simulink model "LC62_PIDControl_V6"  (R2022b)
settings: Solver=ode4  StartTime=0.0  StopTime=SimTime  FixedStep=1/500  RelTol=1e-3
model workspace (MAT data in the model file):
  Tr = 0.1
  freq = 0.002
  hover_w = 0.55
values from neighbouring files (symbols this model uses):
  b = 1.1    [initfun.m]
  c = 0.551    [initfun.m]
  Cll_beta = -0.0518    [initfun.m]
  Cll_del_A = -0.0369 * 5    (= -0.1845)    [initfun.m]
  Cll_del_R = 0.0026    [initfun.m]
  Cll_p = -0.4624    [initfun.m]
  Cll_r = 0.0218    [initfun.m]
  Cm_del_A = 0.001156    [initfun.m]
  Cm_del_E = -0.676    [initfun.m]
  Cn_beta = 0.0866    [initfun.m]
  Cn_del_A = -0.000385    [initfun.m]
  Cn_del_R = -0.0190    (= -0.019)    [initfun.m]
  Cn_p = -0.0048    [initfun.m]
  Cn_r = -0.0723    [initfun.m]
  Cy_beta = -1.1269    [initfun.m]
  Cy_del_R = 0.0534    [initfun.m]
  Cy_p = 0.0    (= 0)    [initfun.m]
  Cy_r = 0.2374    [initfun.m]
  d = 0.849    [initfun.m]
  dx1 = 0.9325+0.049    (= 0.9815)    [initfun.m]
  dx2 = 0.0725-0.049    (= 0.0235)    [initfun.m]
  dx3 = 1.1725-0.049    (= 1.1235)    [initfun.m]
  dy1 = 0.717 + temp_y    (= 0.717)    [initfun.m]
  dy2 = 0.717 - temp_y    (= 0.717)    [initfun.m]
  g = 9.81    [initfun.m]
  m = 41.97    [initfun.m]
  S = S1 + S2    (= 0.8522)    [initfun.m]
  S2 = 0.5898    [initfun.m]
undefined symbols (not defined in the file or in its folder): d2r, Earth, F, Light, MIL, sigbuilder_block, WGS84
libraries: simulink_extras x50, slpidlib x14, simulink x11, dspstat3 x5, aerolibwind2 x3, sharedTrackingLibrary x2, aerolibasang x2, aerolibtransform2 x2, robotcorelib x1, uavutilslib x1, uavalgslib x1, aerolibnav x1
(part 3 of 4)

== system LC62_PIDControl_V6/Position and Acceleration Control/Position Control ==
  note: [ States ]
      | u v w [m/s]
      | phi theta psi [rad]
      | p q r [rad/s]
      | X Y Z [m]
      | U V W [m/s]
  Position cmd : Inport
  States : Inport  Port=2
  Add : Sum  Inputs=+-
  Demux : Demux  Outputs=3
  Mux : Mux  Inputs=3
  PID_X : slpidlib/PID Controller  Controller=PID  Form=Parallel  TimeDomain=Discrete-time  UseExternalTs=off  SampleTime=-1  IntegratorMethod=Forward Euler  FilterMethod=Forward Euler  ControllerParametersSource=internal  P=0.45  I=0.005  UseKiTs=off  D=0.8  N=100  UseFilter=on  TunerSelectOption=Transfer Function Based (PID Tuner App)  InitialConditionSource=internal  InitialConditionForIntegrator=0  InitialConditionForFilter=0  DifferentiatorICPrevScaledInput=0  ExternalReset=none  TrackingMode=off  Kt=1  LimitOutput=on  SatLimitsSource=internal  UpperSaturationLimit=3  LowerSaturationLimit=-3  LinearizeAsGain=on  AntiWindupMode=clamping  Kb=1  LimitIntegrator=off  UpperIntegratorSaturationLimit=inf  LowerIntegratorSaturationLimit=-inf  POutMin=[]  POutMax=[]  IOutMin=[]  IOutMax=[]  DOutMin=[]  DOutMax=[]  NOutMin=[]  NOutMax=[]  SumOutMin=[]  SumOutMax=[]  SaturationOutMin=[]  SaturationOutMax=[]  PParamMin=[]  PParamMax=[]  IParamMin=[]  IParamMax=[]  DParamMin=[]  DParamMax=[]  NParamMin=[]  NParamMax=[]  KbParamMin=[]  KbParamMax=[]  KtParamMin=[]  KtParamMax=[]  KbOutMin=[]  KbOutMax=[]  KtOutMin=[]  KtOutMax=[]  IntegratorOutMin=[]  IntegratorOutMax=[]  FilterOutMin=[]  FilterOutMax=[]  SumI1OutMin=SumI1OutMin  SumI1OutMax=SumI1OutMax  SumI2OutMin=[]  SumI2OutMax=[]  SumI3OutMin=[]  SumI3OutMax=[]  SumI4OutMin=[]  SumI4OutMax=[]  SumDOutMin=[]  SumDOutMax=[]  DifferentiatorOutMin=[]  DifferentiatorOutMax=[]  FilterDiffOutCoefMin=[]  FilterDiffOutCoefMax=[]  ReciprocalOutMin=[]  ReciprocalOutMax=[]  SumDenOutMin=[]  SumDenOutMax=[]  SumNumOutMin=[]  SumNumOutMax=[]  DivideOutMin=[]  DivideOutMax=[]  UdiffTsProdOutMin=[]  UdiffTsProdOutMax=[]  NTsProdOutMin=[]  NTsProdOutMax=[]  UintegralTsProdOutMin=[]  UintegralTsProdOutMax=[]  UngainTsProdOutMin=[]  UngainTsProdOutMax=[]  ClampingZeroOutDataTypeStr=Inherit: Inherit via back propagation  ClampingZeroOutMin=[]  ClampingZeroOutMax=[]  FilterDenConstantOutDataTypeStr=Inherit: Inherit via back propagation  FilterDenConstantOutMin=[]  FilterDenConstantOutMax=[]  PCopyOutDataTypeStr=Inherit: Inherit via back propagation  PCopyOutMin=[]  PCopyOutMax=[]  NCopyOutDataTypeStr=Inherit: Inherit via back propagation  NCopyOutMin=[]  NCopyOutMax=[]  IntegratorContinuousStateAttributes=''  IntegratorStateMustResolveToSignalObject=off  IntegratorRTWStateStorageClass=Auto  FilterContinuousStateAttributes=''  FilterStateMustResolveToSignalObject=off  FilterRTWStateStorageClass=Auto  ParallelPVariant=InternalParameters  IdealPVariant=Disabled  IVariant=InternalParameters  DVariant=InternalParameters  IntegratorVariant=Discrete  SatVariant=Enabled  AWVariant=DiscClampingParallel  PCopyVariant=Disabled  TRVariant=Disabled  FdbkBlocksVariant=Forward  IdealPFdbkVariant=Disabled  SatFdbkVariant=Disabled  DerivativeFilterVariant=ForwardEulerFilter  NVariant=InternalParameters  NCopyVariant=Disabled  FilterICVariant=InternalICsFilter  IntegratorICVariant=InternalICs  ExternalResetVariant=Disabled  TRSumVariant=Passthrough  SumFdbkVariant=Disabled  SumVariant=Sum_PID  TsampFilterVariant=InternalTs  TsampNgainVariant=Passthrough  TsampIntegralVariant=Passthrough  ExternalSaturationOutDataTypeStr=Inherit: Same as second input
      settings: AttributesFormatString=P: %<P>, I: %<I>, D:%<D>
  PID_Y : slpidlib/PID Controller  Controller=PID  Form=Parallel  TimeDomain=Discrete-time  UseExternalTs=off  SampleTime=-1  IntegratorMethod=Forward Euler  FilterMethod=Forward Euler  ControllerParametersSource=internal  P=0.45  I=0.005  UseKiTs=off  D=0.8  N=100  UseFilter=on  TunerSelectOption=Transfer Function Based (PID Tuner App)  InitialConditionSource=internal  InitialConditionForIntegrator=0  InitialConditionForFilter=0  DifferentiatorICPrevScaledInput=0  ExternalReset=none  TrackingMode=off  Kt=1  LimitOutput=on  SatLimitsSource=internal  UpperSaturationLimit=3  LowerSaturationLimit=-3  LinearizeAsGain=on  AntiWindupMode=clamping  Kb=1  LimitIntegrator=off  UpperIntegratorSaturationLimit=inf  LowerIntegratorSaturationLimit=-inf  POutMin=[]  POutMax=[]  IOutMin=[]  IOutMax=[]  DOutMin=[]  DOutMax=[]  NOutMin=[]  NOutMax=[]  SumOutMin=[]  SumOutMax=[]  SaturationOutMin=[]  SaturationOutMax=[]  PParamMin=[]  PParamMax=[]  IParamMin=[]  IParamMax=[]  DParamMin=[]  DParamMax=[]  NParamMin=[]  NParamMax=[]  KbParamMin=[]  KbParamMax=[]  KtParamMin=[]  KtParamMax=[]  KbOutMin=[]  KbOutMax=[]  KtOutMin=[]  KtOutMax=[]  IntegratorOutMin=[]  IntegratorOutMax=[]  FilterOutMin=[]  FilterOutMax=[]  SumI1OutMin=SumI1OutMin  SumI1OutMax=SumI1OutMax  SumI2OutMin=[]  SumI2OutMax=[]  SumI3OutMin=[]  SumI3OutMax=[]  SumI4OutMin=[]  SumI4OutMax=[]  SumDOutMin=[]  SumDOutMax=[]  DifferentiatorOutMin=[]  DifferentiatorOutMax=[]  FilterDiffOutCoefMin=[]  FilterDiffOutCoefMax=[]  ReciprocalOutMin=[]  ReciprocalOutMax=[]  SumDenOutMin=[]  SumDenOutMax=[]  SumNumOutMin=[]  SumNumOutMax=[]  DivideOutMin=[]  DivideOutMax=[]  UdiffTsProdOutMin=[]  UdiffTsProdOutMax=[]  NTsProdOutMin=[]  NTsProdOutMax=[]  UintegralTsProdOutMin=[]  UintegralTsProdOutMax=[]  UngainTsProdOutMin=[]  UngainTsProdOutMax=[]  ClampingZeroOutDataTypeStr=Inherit: Inherit via back propagation  ClampingZeroOutMin=[]  ClampingZeroOutMax=[]  FilterDenConstantOutDataTypeStr=Inherit: Inherit via back propagation  FilterDenConstantOutMin=[]  FilterDenConstantOutMax=[]  PCopyOutDataTypeStr=Inherit: Inherit via back propagation  PCopyOutMin=[]  PCopyOutMax=[]  NCopyOutDataTypeStr=Inherit: Inherit via back propagation  NCopyOutMin=[]  NCopyOutMax=[]  IntegratorContinuousStateAttributes=''  IntegratorStateMustResolveToSignalObject=off  IntegratorRTWStateStorageClass=Auto  FilterContinuousStateAttributes=''  FilterStateMustResolveToSignalObject=off  FilterRTWStateStorageClass=Auto  ParallelPVariant=InternalParameters  IdealPVariant=Disabled  IVariant=InternalParameters  DVariant=InternalParameters  IntegratorVariant=Discrete  SatVariant=Enabled  AWVariant=DiscClampingParallel  PCopyVariant=Disabled  TRVariant=Disabled  FdbkBlocksVariant=Forward  IdealPFdbkVariant=Disabled  SatFdbkVariant=Disabled  DerivativeFilterVariant=ForwardEulerFilter  NVariant=InternalParameters  NCopyVariant=Disabled  FilterICVariant=InternalICsFilter  IntegratorICVariant=InternalICs  ExternalResetVariant=Disabled  TRSumVariant=Passthrough  SumFdbkVariant=Disabled  SumVariant=Sum_PID  TsampFilterVariant=InternalTs  TsampNgainVariant=Passthrough  TsampIntegralVariant=Passthrough  ExternalSaturationOutDataTypeStr=Inherit: Same as second input
      settings: AttributesFormatString=P: %<P>, I: %<I>, D:%<D>
  PID_Z : slpidlib/PID Controller  Controller=PID  Form=Parallel  TimeDomain=Discrete-time  UseExternalTs=off  SampleTime=-1  IntegratorMethod=Forward Euler  FilterMethod=Forward Euler  ControllerParametersSource=internal  P=6.8  I=0  UseKiTs=off  D=2.5  N=14.495  UseFilter=on  TunerSelectOption=Transfer Function Based (PID Tuner App)  InitialConditionSource=internal  InitialConditionForIntegrator=0  InitialConditionForFilter=0  DifferentiatorICPrevScaledInput=0  ExternalReset=none  TrackingMode=off  Kt=1  LimitOutput=on  SatLimitsSource=internal  UpperSaturationLimit=3  LowerSaturationLimit=-3  LinearizeAsGain=on  AntiWindupMode=clamping  Kb=1  LimitIntegrator=off  UpperIntegratorSaturationLimit=inf  LowerIntegratorSaturationLimit=-inf  POutMin=[]  POutMax=[]  IOutMin=[]  IOutMax=[]  DOutMin=[]  DOutMax=[]  NOutMin=[]  NOutMax=[]  SumOutMin=[]  SumOutMax=[]  SaturationOutMin=[]  SaturationOutMax=[]  PParamMin=[]  PParamMax=[]  IParamMin=[]  IParamMax=[]  DParamMin=[]  DParamMax=[]  NParamMin=[]  NParamMax=[]  KbParamMin=[]  KbParamMax=[]  KtParamMin=[]  KtParamMax=[]  KbOutMin=[]  KbOutMax=[]  KtOutMin=[]  KtOutMax=[]  IntegratorOutMin=[]  IntegratorOutMax=[]  FilterOutMin=[]  FilterOutMax=[]  SumI1OutMin=SumI1OutMin  SumI1OutMax=SumI1OutMax  SumI2OutMin=[]  SumI2OutMax=[]  SumI3OutMin=[]  SumI3OutMax=[]  SumI4OutMin=[]  SumI4OutMax=[]  SumDOutMin=[]  SumDOutMax=[]  DifferentiatorOutMin=[]  DifferentiatorOutMax=[]  FilterDiffOutCoefMin=[]  FilterDiffOutCoefMax=[]  ReciprocalOutMin=[]  ReciprocalOutMax=[]  SumDenOutMin=[]  SumDenOutMax=[]  SumNumOutMin=[]  SumNumOutMax=[]  DivideOutMin=[]  DivideOutMax=[]  UdiffTsProdOutMin=[]  UdiffTsProdOutMax=[]  NTsProdOutMin=[]  NTsProdOutMax=[]  UintegralTsProdOutMin=[]  UintegralTsProdOutMax=[]  UngainTsProdOutMin=[]  UngainTsProdOutMax=[]  ClampingZeroOutDataTypeStr=Inherit: Inherit via back propagation  ClampingZeroOutMin=[]  ClampingZeroOutMax=[]  FilterDenConstantOutDataTypeStr=Inherit: Inherit via back propagation  FilterDenConstantOutMin=[]  FilterDenConstantOutMax=[]  PCopyOutDataTypeStr=Inherit: Inherit via back propagation  PCopyOutMin=[]  PCopyOutMax=[]  NCopyOutDataTypeStr=Inherit: Inherit via back propagation  NCopyOutMin=[]  NCopyOutMax=[]  IntegratorContinuousStateAttributes=''  IntegratorStateMustResolveToSignalObject=off  IntegratorRTWStateStorageClass=Auto  FilterContinuousStateAttributes=''  FilterStateMustResolveToSignalObject=off  FilterRTWStateStorageClass=Auto  ParallelPVariant=InternalParameters  IdealPVariant=Disabled  IVariant=InternalParameters  DVariant=InternalParameters  IntegratorVariant=Discrete  SatVariant=Enabled  AWVariant=DiscClampingParallel  PCopyVariant=Disabled  TRVariant=Disabled  FdbkBlocksVariant=Forward  IdealPFdbkVariant=Disabled  SatFdbkVariant=Disabled  DerivativeFilterVariant=ForwardEulerFilter  NVariant=InternalParameters  NCopyVariant=Disabled  FilterICVariant=InternalICsFilter  IntegratorICVariant=InternalICs  ExternalResetVariant=Disabled  TRSumVariant=Passthrough  SumFdbkVariant=Disabled  SumVariant=Sum_PID  TsampFilterVariant=InternalTs  TsampNgainVariant=Passthrough  TsampIntegralVariant=Passthrough  ExternalSaturationOutDataTypeStr=Inherit: Same as second input
      settings: AttributesFormatString=P: %<P>, I: %<I>, D:%<D>
  Selector : Selector  InputPortWidth=15  IndexOptions=Index vector (dialog)  Indices=[10 11 12]  OutputSizes=1
  Selector1 : Selector  InputPortWidth=4  IndexOptions=Index vector (dialog)  Indices=[1 2 3]  OutputSizes=1
  Velocity Cmd : Outport
  tag scope: U_ref_pid=global, V_ref_pid=global
  wires:
  States/1 -> Selector/1
  Position cmd/1 -> Selector1/1
  Selector/1 -> Add/2
  Selector1/1 -> Add/1
  Add/1 -> Demux/1
  Demux/1 -> PID_X/1
  PID_X/1 -> [U_ref_pid], Mux/1
  PID_Z/1 -> Mux/3
  Demux/3 -> PID_Z/1
  PID_Y/1 -> [V_ref_pid], Mux/2
  Demux/2 -> PID_Y/1
  Mux/1 -> Velocity Cmd/1

== system LC62_PIDControl_V6/Position and Acceleration Control/Velocity Control ==
  note: [ States ]
      | u v w [m/s]
      | phi theta psi [rad]
      | p q r [rad/s]
      | X Y Z [m]
      | U V W [m/s]
  Velocity Cmd : Inport
  States : Inport  Port=2
  Add : Sum  Inputs=+-
  Data Type Conversion{,1..5} (6 alike) : DataTypeConversion  OutDataTypeStr=single  SaturateOnIntegerOverflow=off  RndMeth=Floor
  Demux : Demux  Outputs=3
  Mux : Mux  Inputs=3
  PID_Vx : slpidlib/PID Controller  Controller=PID  Form=Parallel  TimeDomain=Discrete-time  UseExternalTs=off  SampleTime=-1  IntegratorMethod=Forward Euler  FilterMethod=Forward Euler  ControllerParametersSource=internal  P=0.35  I=0  UseKiTs=off  D=0.1  N=10  UseFilter=on  TunerSelectOption=Transfer Function Based (PID Tuner App)  InitialConditionSource=internal  InitialConditionForIntegrator=0  InitialConditionForFilter=0  DifferentiatorICPrevScaledInput=0  ExternalReset=none  TrackingMode=off  Kt=1  LimitOutput=on  SatLimitsSource=internal  UpperSaturationLimit=1  LowerSaturationLimit=-1  LinearizeAsGain=on  AntiWindupMode=clamping  Kb=1  LimitIntegrator=off  UpperIntegratorSaturationLimit=inf  LowerIntegratorSaturationLimit=-inf  PGainOutDataTypeStr=single  PProdOutDataTypeStr=single  POutMin=[]  POutMax=[]  IGainOutDataTypeStr=single  IProdOutDataTypeStr=single  IOutMin=[]  IOutMax=[]  DGainOutDataTypeStr=single  DProdOutDataTypeStr=single  DOutMin=[]  DOutMax=[]  NGainOutDataTypeStr=single  NProdOutDataTypeStr=single  NOutMin=[]  NOutMax=[]  SumOutDataTypeStr=single  SumOutMin=[]  SumOutMax=[]  SaturationOutDataTypeStr=single  SaturationOutMin=[]  SaturationOutMax=[]  PParamMin=[]  PParamMax=[]  IParamMin=[]  IParamMax=[]  DParamMin=[]  DParamMax=[]  NParamMin=[]  NParamMax=[]  KbParamMin=[]  KbParamMax=[]  KtParamMin=[]  KtParamMax=[]  KbOutMin=[]  KbOutMax=[]  KtOutMin=[]  KtOutMax=[]  IntegratorOutMin=[]  IntegratorOutMax=[]  FilterOutMin=[]  FilterOutMax=[]  SumI1OutMin=SumI1OutMin  SumI1OutMax=SumI1OutMax  SumI2OutMin=[]  SumI2OutMax=[]  SumI3OutMin=[]  SumI3OutMax=[]  SumI4OutMin=[]  SumI4OutMax=[]  SumDOutMin=[]  SumDOutMax=[]  DifferentiatorOutMin=[]  DifferentiatorOutMax=[]  FilterDiffOutCoefMin=[]  FilterDiffOutCoefMax=[]  ReciprocalOutMin=[]  ReciprocalOutMax=[]  SumDenOutMin=[]  SumDenOutMax=[]  SumNumOutMin=[]  SumNumOutMax=[]  DivideOutMin=[]  DivideOutMax=[]  UdiffTsProdOutMin=[]  UdiffTsProdOutMax=[]  NTsProdOutMin=[]  NTsProdOutMax=[]  UintegralTsProdOutMin=[]  UintegralTsProdOutMax=[]  UngainTsProdOutMin=[]  UngainTsProdOutMax=[]  ClampingZeroOutDataTypeStr=Inherit: Inherit via back propagation  ClampingZeroOutMin=[]  ClampingZeroOutMax=[]  FilterDenConstantOutDataTypeStr=Inherit: Inherit via back propagation  FilterDenConstantOutMin=[]  FilterDenConstantOutMax=[]  PCopyOutDataTypeStr=Inherit: Inherit via back propagation  PCopyOutMin=[]  PCopyOutMax=[]  NCopyOutDataTypeStr=Inherit: Inherit via back propagation  NCopyOutMin=[]  NCopyOutMax=[]  IntegratorContinuousStateAttributes=''  IntegratorStateMustResolveToSignalObject=off  IntegratorRTWStateStorageClass=Auto  FilterContinuousStateAttributes=''  FilterStateMustResolveToSignalObject=off  FilterRTWStateStorageClass=Auto  ParallelPVariant=InternalParameters  IdealPVariant=Disabled  IVariant=InternalParameters  DVariant=InternalParameters  IntegratorVariant=Discrete  SatVariant=Enabled  AWVariant=DiscClampingParallel  PCopyVariant=Disabled  TRVariant=Disabled  FdbkBlocksVariant=Forward  IdealPFdbkVariant=Disabled  SatFdbkVariant=Disabled  DerivativeFilterVariant=ForwardEulerFilter  NVariant=InternalParameters  NCopyVariant=Disabled  FilterICVariant=InternalICsFilter  IntegratorICVariant=InternalICs  ExternalResetVariant=Disabled  TRSumVariant=Passthrough  SumFdbkVariant=Disabled  SumVariant=Sum_PID  TsampFilterVariant=InternalTs  TsampNgainVariant=Passthrough  TsampIntegralVariant=Passthrough  ExternalSaturationOutDataTypeStr=Inherit: Same as second input
      settings: AttributesFormatString=P: %<P>, I: %<I>, D:%<D>
  PID_Vy : slpidlib/PID Controller  Controller=PID  Form=Parallel  TimeDomain=Discrete-time  UseExternalTs=off  SampleTime=-1  IntegratorMethod=Forward Euler  FilterMethod=Forward Euler  ControllerParametersSource=internal  P=0.35  I=0  UseKiTs=off  D=0.1  N=10  UseFilter=on  TunerSelectOption=Transfer Function Based (PID Tuner App)  InitialConditionSource=internal  InitialConditionForIntegrator=0  InitialConditionForFilter=0  DifferentiatorICPrevScaledInput=0  ExternalReset=none  TrackingMode=off  Kt=1  LimitOutput=on  SatLimitsSource=internal  UpperSaturationLimit=1  LowerSaturationLimit=-1  LinearizeAsGain=on  AntiWindupMode=clamping  Kb=1  LimitIntegrator=off  UpperIntegratorSaturationLimit=inf  LowerIntegratorSaturationLimit=-inf  POutMin=[]  POutMax=[]  IOutMin=[]  IOutMax=[]  DOutMin=[]  DOutMax=[]  NOutMin=[]  NOutMax=[]  SumOutMin=[]  SumOutMax=[]  SaturationOutMin=[]  SaturationOutMax=[]  PParamMin=[]  PParamMax=[]  IParamMin=[]  IParamMax=[]  DParamMin=[]  DParamMax=[]  NParamMin=[]  NParamMax=[]  KbParamMin=[]  KbParamMax=[]  KtParamMin=[]  KtParamMax=[]  KbOutMin=[]  KbOutMax=[]  KtOutMin=[]  KtOutMax=[]  IntegratorOutMin=[]  IntegratorOutMax=[]  FilterOutMin=[]  FilterOutMax=[]  SumI1OutMin=SumI1OutMin  SumI1OutMax=SumI1OutMax  SumI2OutMin=[]  SumI2OutMax=[]  SumI3OutMin=[]  SumI3OutMax=[]  SumI4OutMin=[]  SumI4OutMax=[]  SumDOutMin=[]  SumDOutMax=[]  DifferentiatorOutMin=[]  DifferentiatorOutMax=[]  FilterDiffOutCoefMin=[]  FilterDiffOutCoefMax=[]  ReciprocalOutMin=[]  ReciprocalOutMax=[]  SumDenOutMin=[]  SumDenOutMax=[]  SumNumOutMin=[]  SumNumOutMax=[]  DivideOutMin=[]  DivideOutMax=[]  UdiffTsProdOutMin=[]  UdiffTsProdOutMax=[]  NTsProdOutMin=[]  NTsProdOutMax=[]  UintegralTsProdOutMin=[]  UintegralTsProdOutMax=[]  UngainTsProdOutMin=[]  UngainTsProdOutMax=[]  ClampingZeroOutDataTypeStr=Inherit: Inherit via back propagation  ClampingZeroOutMin=[]  ClampingZeroOutMax=[]  FilterDenConstantOutDataTypeStr=Inherit: Inherit via back propagation  FilterDenConstantOutMin=[]  FilterDenConstantOutMax=[]  PCopyOutDataTypeStr=Inherit: Inherit via back propagation  PCopyOutMin=[]  PCopyOutMax=[]  NCopyOutDataTypeStr=Inherit: Inherit via back propagation  NCopyOutMin=[]  NCopyOutMax=[]  IntegratorContinuousStateAttributes=''  IntegratorStateMustResolveToSignalObject=off  IntegratorRTWStateStorageClass=Auto  FilterContinuousStateAttributes=''  FilterStateMustResolveToSignalObject=off  FilterRTWStateStorageClass=Auto  ParallelPVariant=InternalParameters  IdealPVariant=Disabled  IVariant=InternalParameters  DVariant=InternalParameters  IntegratorVariant=Discrete  SatVariant=Enabled  AWVariant=DiscClampingParallel  PCopyVariant=Disabled  TRVariant=Disabled  FdbkBlocksVariant=Forward  IdealPFdbkVariant=Disabled  SatFdbkVariant=Disabled  DerivativeFilterVariant=ForwardEulerFilter  NVariant=InternalParameters  NCopyVariant=Disabled  FilterICVariant=InternalICsFilter  IntegratorICVariant=InternalICs  ExternalResetVariant=Disabled  TRSumVariant=Passthrough  SumFdbkVariant=Disabled  SumVariant=Sum_PID  TsampFilterVariant=InternalTs  TsampNgainVariant=Passthrough  TsampIntegralVariant=Passthrough  ExternalSaturationOutDataTypeStr=Inherit: Same as second input
      settings: AttributesFormatString=P: %<P>, I: %<I>, D:%<D>
  PID_Vz : slpidlib/PID Controller  Controller=PID  Form=Parallel  TimeDomain=Discrete-time  UseExternalTs=off  SampleTime=-1  IntegratorMethod=Forward Euler  FilterMethod=Forward Euler  ControllerParametersSource=internal  P=6.8  I=0  UseKiTs=off  D=2.5  N=14.495  UseFilter=on  TunerSelectOption=Transfer Function Based (PID Tuner App)  InitialConditionSource=internal  InitialConditionForIntegrator=0  InitialConditionForFilter=0  DifferentiatorICPrevScaledInput=0  ExternalReset=none  TrackingMode=off  Kt=1  LimitOutput=on  SatLimitsSource=internal  UpperSaturationLimit=2  LowerSaturationLimit=-2  LinearizeAsGain=on  AntiWindupMode=clamping  Kb=1  LimitIntegrator=off  UpperIntegratorSaturationLimit=inf  LowerIntegratorSaturationLimit=-inf  POutMin=[]  POutMax=[]  IOutMin=[]  IOutMax=[]  DOutMin=[]  DOutMax=[]  NOutMin=[]  NOutMax=[]  SumOutMin=[]  SumOutMax=[]  SaturationOutMin=[]  SaturationOutMax=[]  PParamMin=[]  PParamMax=[]  IParamMin=[]  IParamMax=[]  DParamMin=[]  DParamMax=[]  NParamMin=[]  NParamMax=[]  KbParamMin=[]  KbParamMax=[]  KtParamMin=[]  KtParamMax=[]  KbOutMin=[]  KbOutMax=[]  KtOutMin=[]  KtOutMax=[]  IntegratorOutMin=[]  IntegratorOutMax=[]  FilterOutMin=[]  FilterOutMax=[]  SumI1OutMin=SumI1OutMin  SumI1OutMax=SumI1OutMax  SumI2OutMin=[]  SumI2OutMax=[]  SumI3OutMin=[]  SumI3OutMax=[]  SumI4OutMin=[]  SumI4OutMax=[]  SumDOutMin=[]  SumDOutMax=[]  DifferentiatorOutMin=[]  DifferentiatorOutMax=[]  FilterDiffOutCoefMin=[]  FilterDiffOutCoefMax=[]  ReciprocalOutMin=[]  ReciprocalOutMax=[]  SumDenOutMin=[]  SumDenOutMax=[]  SumNumOutMin=[]  SumNumOutMax=[]  DivideOutMin=[]  DivideOutMax=[]  UdiffTsProdOutMin=[]  UdiffTsProdOutMax=[]  NTsProdOutMin=[]  NTsProdOutMax=[]  UintegralTsProdOutMin=[]  UintegralTsProdOutMax=[]  UngainTsProdOutMin=[]  UngainTsProdOutMax=[]  ClampingZeroOutDataTypeStr=Inherit: Inherit via back propagation  ClampingZeroOutMin=[]  ClampingZeroOutMax=[]  FilterDenConstantOutDataTypeStr=Inherit: Inherit via back propagation  FilterDenConstantOutMin=[]  FilterDenConstantOutMax=[]  PCopyOutDataTypeStr=Inherit: Inherit via back propagation  PCopyOutMin=[]  PCopyOutMax=[]  NCopyOutDataTypeStr=Inherit: Inherit via back propagation  NCopyOutMin=[]  NCopyOutMax=[]  IntegratorContinuousStateAttributes=''  IntegratorStateMustResolveToSignalObject=off  IntegratorRTWStateStorageClass=Auto  FilterContinuousStateAttributes=''  FilterStateMustResolveToSignalObject=off  FilterRTWStateStorageClass=Auto  ParallelPVariant=InternalParameters  IdealPVariant=Disabled  IVariant=InternalParameters  DVariant=InternalParameters  IntegratorVariant=Discrete  SatVariant=Enabled  AWVariant=DiscClampingParallel  PCopyVariant=Disabled  TRVariant=Disabled  FdbkBlocksVariant=Forward  IdealPFdbkVariant=Disabled  SatFdbkVariant=Disabled  DerivativeFilterVariant=ForwardEulerFilter  NVariant=InternalParameters  NCopyVariant=Disabled  FilterICVariant=InternalICsFilter  IntegratorICVariant=InternalICs  ExternalResetVariant=Disabled  TRSumVariant=Passthrough  SumFdbkVariant=Disabled  SumVariant=Sum_PID  TsampFilterVariant=InternalTs  TsampNgainVariant=Passthrough  TsampIntegralVariant=Passthrough  ExternalSaturationOutDataTypeStr=Inherit: Same as second input
      settings: AttributesFormatString=P: %<P>, I: %<I>, D:%<D>
  Selector : Selector  InputPortWidth=15  IndexOptions=Index vector (dialog)  Indices=[13 14 15]  OutputSizes=1
  Accel Cmd : Outport
  wires:
  States/1 -> Selector/1
  Selector/1 -> Add/2
  Velocity Cmd/1 -> Add/1
  Add/1 -> Demux/1
  Mux/1 -> Accel Cmd/1
  Demux/3 -> Data Type Conversion5/1
  Demux/2 -> Data Type Conversion3/1
  Data Type Conversion3/1 -> PID_Vy/1
  PID_Vy/1 -> Data Type Conversion1/1
  Data Type Conversion1/1 -> Mux/2
  Data Type Conversion/1 -> Mux/3
  PID_Vz/1 -> Data Type Conversion/1
  Data Type Conversion5/1 -> PID_Vz/1
  Demux/1 -> Data Type Conversion4/1
  Data Type Conversion4/1 -> PID_Vx/1
  PID_Vx/1 -> Data Type Conversion2/1
  Data Type Conversion2/1 -> Mux/1

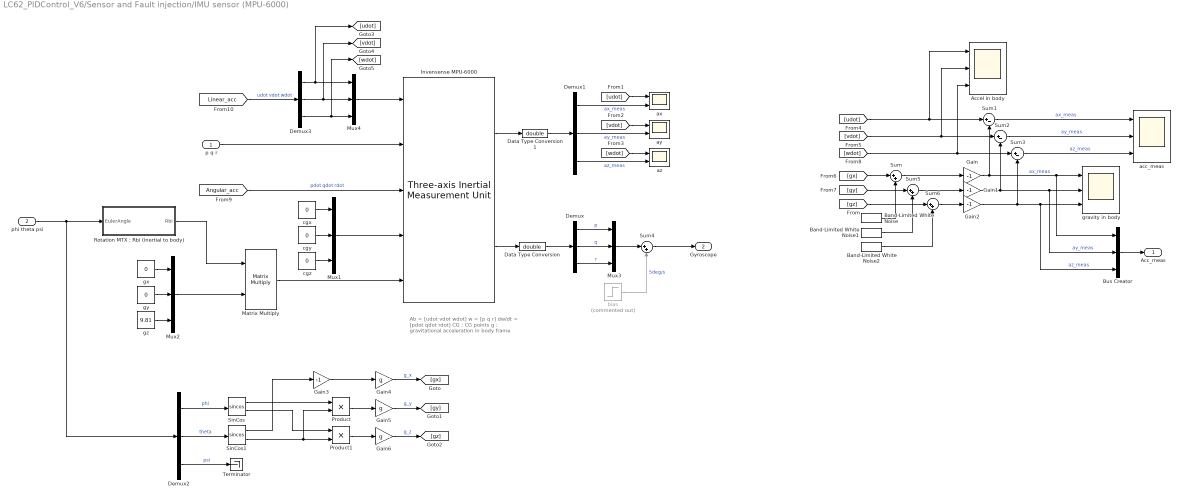
== system LC62_PIDControl_V6/Sensor and Fault injection/IMU sensor (MPU-6000) ==
  note: Ab = [udot vdot wdot]
      | w = [p q r]
      | dw/dt = [pdot qdot rdot]
      | CG : CG points
      | g : gravitational acceleration in body frame
  p q r : Inport
  phi theta psi : Inport  Port=2
  Accel in body : Scope  NumInputPorts=3
  Band-Limited White Noise : simulink/Sources/Band-Limited White Noise  Cov=[1e-7]  Ts=1/freq  seed=[348631]
  Band-Limited White Noise1 : simulink/Sources/Band-Limited White Noise  Cov=[1e-7]  Ts=1/freq  seed=[366719]
  Band-Limited White Noise2 : simulink/Sources/Band-Limited White Noise  Cov=[1e-7]  Ts=1/freq  seed=[978432]
  Bus Creator : BusCreator  Inputs=3
  Data Type Conversion : DataTypeConversion  OutDataTypeStr=double  SaturateOnIntegerOverflow=off  RndMeth=Floor
  Data Type Conversion1 : DataTypeConversion  OutDataTypeStr=double  SaturateOnIntegerOverflow=off  RndMeth=Floor
  Demux{,1..3} (4 alike) : Demux  Outputs=3
  Gain{,1..3} (4 alike) : Gain  Gain=-1
  Gain4 : Gain  Gain=g
  Gain5 : Gain  Gain=g
  Gain6 : Gain  Gain=g
  Invensense MPU-6000 : aerolibnav/Three-axis Inertial Measurement Unit  units=Metric (MKS)  imu=[0 0 0]  i_Ts=1/freq  dtype_a=off  w_a=190  z_a=0.707  a_sf_cc=[0.98 0 0; 0 0.98 0; 0 0 0.98]  a_bias=[0 0 0]  a_sat="[-19.62  -19.62  -19.62 19.62 19.62 19.62]"  dtype_g=off  w_g=190  z_g=0.707  g_sf_cc=[.98 0 0; 0 .98 0; 0 0 .98]  g_bias=[0 0 0]  g_sens=[0 0 0]  g_sat="[-4.36  -4.36  -4.36 4.36 4.36 4.36]"  i_rand=on  i_seeds=[348631 366719 978432 189621 128794 214632]  i_pow=[0.0000001 0.0000001 0.0000001 0.0000000005 0.0000000005 0.0000000005]
  Matrix Multiply : Product  Multiplication=Matrix(*)
  Mux{1..4} (4 alike) : Mux  Inputs=3
  Product : Product
  Product1 : Product
  "Rotation MTX : Rbi (inertial to body)" : MATLAB Function  TreatAsAtomicUnit=on
  SinCos : Trigonometry  Operator=sincos
  SinCos1 : Trigonometry  Operator=sincos
  Sum{,4..6} (4 alike) : Sum  Inputs=|++
  Sum1 : Sum  Inputs=|+-
  Sum2 : Sum  Inputs=|+-
  Sum3 : Sum  Inputs=|+-
  Terminator : Terminator
  acc_meas : Scope  NumInputPorts=3
  ax : Scope  NumInputPorts=2
  ay : Scope  NumInputPorts=2
  az : Scope  NumInputPorts=2
  bias : Step  Commented=on  Time=5  After=5*d2r
  cgx : Constant  Value=0
  cgy : Constant  Value=0
  cgz : Constant  Value=0
  gravity in body : Scope  NumInputPorts=3
  gx : Constant  Value=0
  gy : Constant  Value=0
  gz : Constant  Value=9.81
  Acc_meas : Outport
  Gyroscope : Outport  Port=2
  wires:
  gy/1 -> Mux2/2
  Demux/3 -> Mux3/3  "r"
  Demux/2 -> Mux3/2  "q"
  Demux/1 -> Mux3/1  "p"
  cgy/1 -> Mux1/2
  cgx/1 -> Mux1/1
  cgz/1 -> Mux1/3
  Mux1/1 -> Invensense MPU-6000/4
  Data Type Conversion/1 -> Demux/1
  Matrix Multiply/1 -> Invensense MPU-6000/5
  gz/1 -> Mux2/3
  gx/1 -> Mux2/1
  "Rotation MTX : Rbi (inertial to body)"/1(Rbi) -> Matrix Multiply/1
  Mux2/1 -> Matrix Multiply/2
  [Angular_acc] -> Invensense MPU-6000/3  "pdot qdot rdot"
  p q r/1 -> Invensense MPU-6000/2
  Invensense MPU-6000/1 -> Data Type Conversion1/1
  Invensense MPU-6000/2 -> Data Type Conversion/1
  Sum4/1 -> Gyroscope/1
  Mux3/1 -> Sum4/1
  bias/1 -> Sum4/2  "5deg/s"
  Data Type Conversion1/1 -> Demux1/1
  Demux1/2 -> ay/2  "ay_meas"
  Demux1/3 -> az/2  "az_meas"
  Demux1/1 -> ax/2  "ax_meas"
  [Linear_acc] -> Demux3/1  "udot vdot wdot"
  Mux4/1 -> Invensense MPU-6000/1
  [udot] -> Accel in body/1, Sum1/1
  [vdot] -> Accel in body/2, Sum2/1
  [wdot] -> Accel in body/3, Sum3/1
  Bus Creator/1 -> Acc_meas/1
  Sum3/1 -> acc_meas/3  "az_meas"
  Sum2/1 -> acc_meas/2  "ay_meas"
  Sum1/1 -> acc_meas/1  "ax_meas"
  Demux3/1 -> [udot], Mux4/1
  Demux3/2 -> [vdot], Mux4/2
  Demux3/3 -> [wdot], Mux4/3
  [udot] -> ax/1
  [vdot] -> ay/1
  [wdot] -> az/1
  Gain/1 -> Bus Creator/1, gravity in body/1, Sum1/2  "ax_meas"
  Gain1/1 -> Bus Creator/2, gravity in body/2, Sum2/2  "ay_meas"
  Gain2/1 -> Bus Creator/3, gravity in body/3, Sum3/2  "az_meas"
  [gx] -> Sum/1
  Sum/1 -> Gain/1
  Band-Limited White Noise/1 -> Sum/2
  [gy] -> Sum5/1
  Sum5/1 -> Gain1/1
  Band-Limited White Noise1/1 -> Sum5/2
  Sum6/1 -> Gain2/1
  [gz] -> Sum6/1
  Band-Limited White Noise2/1 -> Sum6/2
  SinCos/2 -> Product1/1
  Demux2/3 -> Terminator/1  "psi"
  SinCos/1 -> Product/1
  Demux2/1 -> SinCos/1  "phi"
  Product/1 -> Gain5/1
  SinCos1/1 -> Gain3/1
  Gain5/1 -> [gy]  "g_y"
  Product1/1 -> Gain6/1
  SinCos1/2 -> Product1/2, Product/2
  Demux2/2 -> SinCos1/1  "theta"
  Gain6/1 -> [gz]  "g_z"
  Gain4/1 -> [gx]  "g_x"
  Gain3/1 -> Gain4/1
  phi theta psi/1 -> "Rotation MTX : Rbi (inertial to body)"/1(EulerAngle), Demux2/1

== system LC62_PIDControl_V6/Sensor and Fault injection/Signal Builder1 ==
  Demux : Demux  Tag=STV Demux  Outputs=1
      settings: DisplayOption=none
  FromWs : FromWorkspace  Tag=STV FromWs  VariableName=tuvar
      SigBuilderData=|
      | common.afterFinalStr = 'Extrapolate'
      | common.sampleTime = 0
      | dataSet.timeRange = [0 30]
      | dataSet.name = 'Group 1'
      | sbobj.Groups.Name = 'Group 1'
      | sbobj.Groups.Signals.Name = 'Signal 1'
      | sbobj.Groups.Signals.XData = [0 2 6 6.5 7 7.5 8 8.5 9 9.5 10 10.5 11 11.5 12 12.5 13 13.5 14 14.5 15 15.5 16 16.5 17 17.5 18 18.5 19 19.5 20 26 28 30]
      | sbobj.Groups.Signals.YData = [0 6.12323399574e-16 6.12323399574e-16 -3.53553390593 -5 -3.53553390593 0 3.53553390593 5 3.53553390593 6.12323399574e-16 -3.53553390593 -5 -3.53553390593 0 3.53553390593 5 3.53553390593 6.12323399574e-16 -3.53553390593 -5 -3.53553390593 0 3.53553390593 5 3.53553390593 6.12323399574e-16 -3.53553390593 -5 -3.53553390593 0 6.12323399574e-16 0 6.12323399574e-16]
      | sbobj.Groups.TimeRange = [0 30]
  Signal 1 : Outport  Tag=STV Outport
  wires:
  FromWs/1 -> Demux/1
  Demux/1 -> Signal 1/1

== system LC62_PIDControl_V6/System Dynamics (LC62-50B)/Faults ==
  note: Note: Fault can be set up between 0 to 1.
      | 1: normal
      | 0: full failure
      | This can be changed by adjusting the equations within the S-function.
  Bus Creator : BusCreator  Inputs=6
  Bus to Vector : BusToVector
  Constant6 : Constant
  Demux : Demux  Outputs=6
  Manual Switch{,1,3..5} (5 alike) : ManualSwitch
  Manual Switch2 : ManualSwitch  CurrentSetting=0
  Mux : Mux  Inputs=6
  Transfer Fcn{,1..5} (6 alike) : TransferFcn  Numerator=1  Denominator=[0.01 1]
  fault at s : Step  Time=50  Before=1  After=0.4  SampleTime=0
  Faults : Outport
  wires:
  Demux/1 -> Transfer Fcn/1
  Manual Switch1/1 -> Bus Creator/2  "motor 2"
  Bus Creator/1 -> Bus to Vector/1
  Mux/1 -> Faults/1
  fault at s/1 -> Manual Switch5/2, Manual Switch2/2, Manual Switch/2, Manual Switch3/2, Manual Switch4/2, Manual Switch1/2
  Manual Switch5/1 -> Bus Creator/1  "motor 1"
  Manual Switch3/1 -> Bus Creator/4  "motor 4"
  Constant6/1 -> Manual Switch5/1, Manual Switch2/1, Manual Switch/1, Manual Switch3/1, Manual Switch4/1, Manual Switch1/1  "motor 1"
  Transfer Fcn2/1 -> Mux/3
  Transfer Fcn4/1 -> Mux/5
  Demux/2 -> Transfer Fcn1/1
  Manual Switch4/1 -> Bus Creator/3  "motor 3"
  Bus to Vector/1 -> Demux/1
  Transfer Fcn/1 -> Mux/1
  Manual Switch/1 -> Bus Creator/5  "motor 5"
  Transfer Fcn3/1 -> Mux/4
  Transfer Fcn1/1 -> Mux/2
  Transfer Fcn5/1 -> Mux/6
  Demux/6 -> Transfer Fcn5/1
  Manual Switch2/1 -> Bus Creator/6  "motor 6"
  Demux/5 -> Transfer Fcn4/1
  Demux/3 -> Transfer Fcn2/1
  Demux/4 -> Transfer Fcn3/1

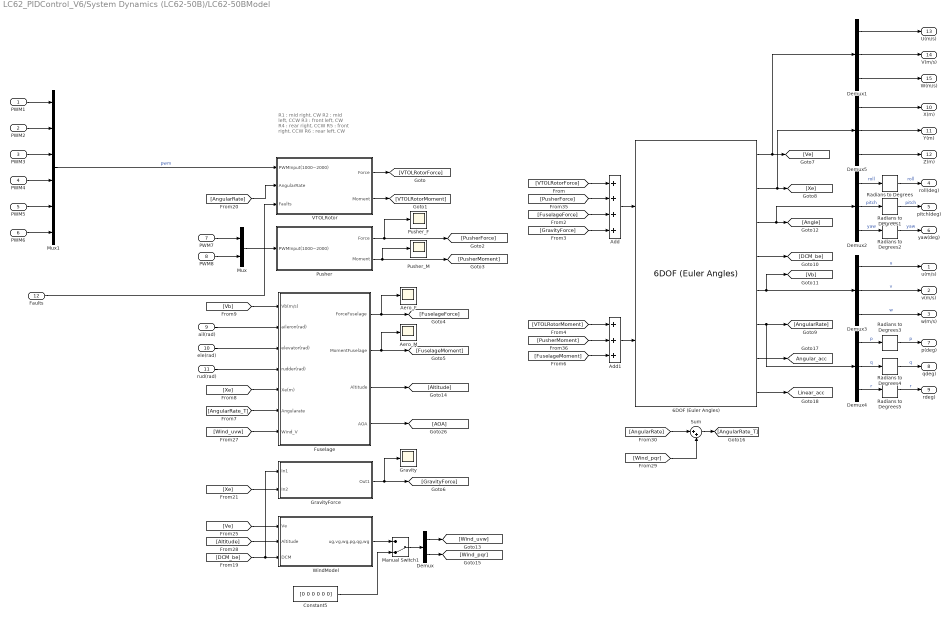
== system LC62_PIDControl_V6/System Dynamics (LC62-50B)/LC62-50BModel ==
  note: R1 : mid right, CW
      | R2 : mid left, CCW
      | R3 : front left, CW
      | R4 : rear right, CCW
      | R5 : front right, CCW
      | R6 : rear left, CW
  PWM1 : Inport
  PWM2 : Inport  Port=2
  PWM3 : Inport  Port=3
  PWM4 : Inport  Port=4
  PWM5 : Inport  Port=5
  PWM6 : Inport  Port=6
  PWM7 : Inport  Port=7
  PWM8 : Inport  Port=8
  ail(rad) : Inport  Port=9
  ele(rad) : Inport  Port=10
  rud(rad) : Inport  Port=11
  Faults : Inport  Port=12
  6DOF (Euler Angles) : shared6dof/6DOF (Euler Angles)  units=Metric (MKS)  mtype=Fixed  rep=Euler Angles  xme_0=[0 0 -10]  Vm_0=[0 0 0]  eul_0=[0 0 0]  pm_0=[0 0 0]  mass_0=m  mass_e=0.5  mass_f=2.0  inertia=InertiaM  inertia_e=eye(3)  inertia_f=2*eye(3)  k_quat=1.0  vre_flag=on  abi_flag=off  aMode=0  xme_statename=''  Vm_statename=''  eul_statename=''  quat_statename=''  pm_statename=''  mass_statename=''
  Add : Sum  Inputs=++++
  Add1 : Sum  Inputs=+++
  Aero_F : Scope
  Aero_M : Scope
  Constant5 : Constant  Value=[0 0 0 0 0 0]
  Demux : Demux  Outputs=2
  Demux{1..5} (5 alike) : Demux  Outputs=3
  Fuselage : Subsystem
  Gravity : Scope
  GravityForce : Subsystem
  Manual Switch1 : ManualSwitch  CurrentSetting=0
  Mux : Mux  Inputs=2
  Mux1 : Mux  Inputs=6
  Pusher : Subsystem
  Pusher_F : Scope
  Pusher_M : Scope
  Radians to Degrees{,1..5} (6 alike) : simulink_extras/Transformations/Radians to Degrees
  Sum : Sum  Inputs=|++
  VTOLRotor : Subsystem
  WindModel : Subsystem
  u(m/s) : Outport
  v(m/s) : Outport  Port=2
  w(m/s) : Outport  Port=3
  roll(deg) : Outport  Port=4
  pitch(deg) : Outport  Port=5
  yaw(deg) : Outport  Port=6
  p(deg) : Outport  Port=7
  qdeg) : Outport  Port=8
  rdeg) : Outport  Port=9
  X(m) : Outport  Port=10
  Y(m) : Outport  Port=11
  Z(m) : Outport  Port=12
  U(m/s) : Outport  Port=13
  V(m/s) : Outport  Port=14
  W(m/s) : Outport  Port=15
  tag scope: Angular_acc=global, Linear_acc=global
  wires:
  VTOLRotor/1(Force) -> [VTOLRotorForce]
  Mux1/1 -> VTOLRotor/1(PWMInput(1000~2000))  "pwm"
  [AngularRate] -> Sum/1
  PWM3/1 -> Mux1/3
  Fuselage/3(Altitude) -> [Altitude]
  WindModel/1(ug,vg,wg,pg,qg,wg) -> Manual Switch1/1
  ail(rad)/1 -> Fuselage/2(aileron(rad))
  6DOF (Euler Angles)/5 -> Demux3/1, [Vb]
  Constant5/1 -> Manual Switch1/2
  Fuselage/4(AOA) -> [AOA]
  ele(rad)/1 -> Fuselage/3(elevator(rad))
  [VTOLRotorMoment] -> Add1/1
  [AngularRate] -> VTOLRotor/2(AngularRate)
  [Wind_uvw] -> Fuselage/7(Wind_V)
  [Vb] -> Fuselage/1(Vb(m/s))
  [AngularRate_T] -> Fuselage/6(Angularate)
  [FuselageMoment] -> Add1/3
  rud(rad)/1 -> Fuselage/4(rudder(rad))
  [VTOLRotorForce] -> Add/1
  [GravityForce] -> Add/4
  VTOLRotor/2(Moment) -> [VTOLRotorMoment]
  [DCM_be] -> WindModel/3(DCM), GravityForce/1(In1)
  [Altitude] -> WindModel/2(Altitude)
  [FuselageForce] -> Add/3
  Demux2/2 -> Radians to Degrees1/1  "pitch"
  GravityForce/1(Out1) -> Gravity/1, [GravityForce]
  Sum/1 -> [AngularRate_T]
  [PusherForce] -> Add/2
  6DOF (Euler Angles)/3 -> [Angle], Demux2/1
  Demux/1 -> [Wind_uvw]
  Add/1 -> 6DOF (Euler Angles)/1
  6DOF (Euler Angles)/4 -> [DCM_be]
  6DOF (Euler Angles)/2 -> Demux5/1, [Xe]
  Demux/2 -> [Wind_pqr]
  PWM2/1 -> Mux1/2
  [PusherMoment] -> Add1/2
  [Ve] -> WindModel/1(Ve)
  Add1/1 -> 6DOF (Euler Angles)/2
  6DOF (Euler Angles)/1 -> [Ve], Demux1/1
  Manual Switch1/1 -> Demux/1
  Fuselage/1(ForceFuselage) -> Aero_F/1, [FuselageForce]
  6DOF (Euler Angles)/6 -> [AngularRate], Demux4/1
  PWM7/1 -> Mux/1
  [Wind_pqr] -> Sum/2
  [Xe] -> Fuselage/5(Xe(m))
  PWM8/1 -> Mux/2
  Demux2/3 -> Radians to Degrees2/1  "yaw"
  Fuselage/2(MomentFuselage) -> [FuselageMoment], Aero_M/1
  [Xe] -> GravityForce/2(In2)
  PWM6/1 -> Mux1/6
  PWM5/1 -> Mux1/5
  PWM1/1 -> Mux1/1
  PWM4/1 -> Mux1/4
  Mux/1 -> Pusher/1(PWMInput(1000~2000))
  Demux3/3 -> w(m/s)/1  "w"
  Demux2/1 -> Radians to Degrees/1  "roll"
  Demux3/2 -> v(m/s)/1  "v"
  Demux3/1 -> u(m/s)/1  "u"
  Demux4/1 -> Radians to Degrees3/1  "p"
  Demux4/2 -> Radians to Degrees4/1  "q"
  Demux4/3 -> Radians to Degrees5/1  "r"
  Pusher/2(Moment) -> Pusher_M/1, [PusherMoment]
  Pusher/1(Force) -> Pusher_F/1, [PusherForce]
  Demux5/3 -> Z(m)/1
  Demux5/2 -> Y(m)/1
  Demux5/1 -> X(m)/1
  Demux1/1 -> U(m/s)/1
  Demux1/2 -> V(m/s)/1
  Demux1/3 -> W(m/s)/1
  Radians to Degrees1/1 -> pitch(deg)/1  "pitch"
  Radians to Degrees/1 -> roll(deg)/1  "roll"
  Radians to Degrees2/1 -> yaw(deg)/1  "yaw"
  Radians to Degrees3/1 -> p(deg)/1  "p"
  Radians to Degrees4/1 -> qdeg)/1  "q"
  Radians to Degrees5/1 -> rdeg)/1  "r"
  6DOF (Euler Angles)/7 -> [Angular_acc]
  6DOF (Euler Angles)/8 -> [Linear_acc]
  Faults/1 -> VTOLRotor/3(Faults)

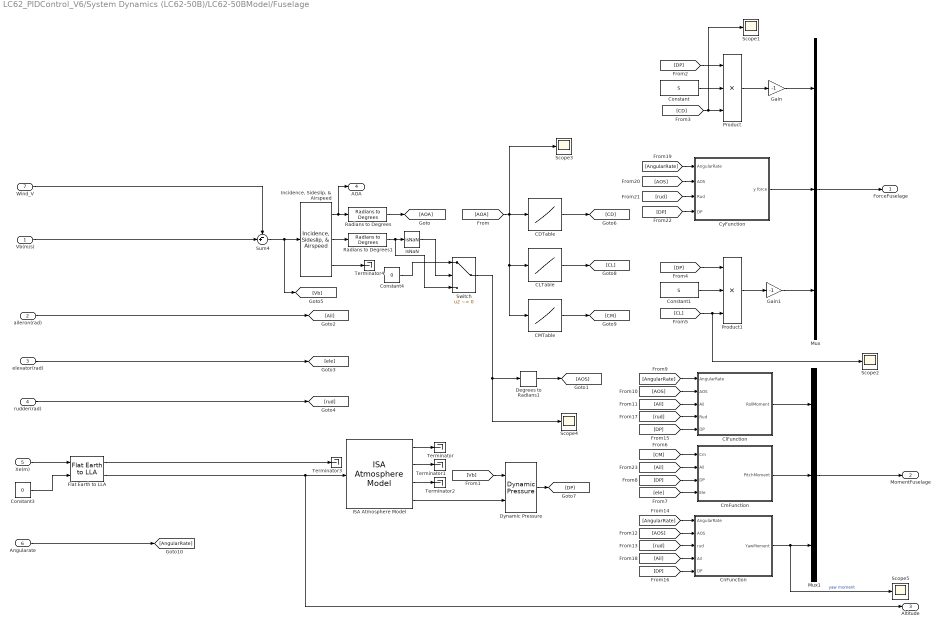
== system LC62_PIDControl_V6/System Dynamics (LC62-50B)/LC62-50BModel/Fuselage ==
  Vb(m/s) : Inport
  aileron(rad) : Inport  Port=2
  elevator(rad) : Inport  Port=3
  rudder(rad) : Inport  Port=4
  Xe(m) : Inport  Port=5
  Angularate : Inport  Port=6
  Wind_V : Inport  Port=7
  CDTable : Lookup_n-D  NumberOfTableDimensions=1  BreakpointsForDimension1=[0, 2, 4, 6, 8, 10, 12, 14, 16]  Table=[0.0617, 0.0668, 0.0788, 0.0948, 0.1199, 0.1504, 0.2105, 0.2594, 0.3128]  ExtrapMethod=Clip  UseLastTableValue=on  InternalRulePriority=Speed  RndMeth=Simplest
  CLTable : Lookup_n-D  NumberOfTableDimensions=1  BreakpointsForDimension1=[0, 2, 4, 6, 8, 10, 12, 14, 16]  Table=[0.1931, 0.4075, 0.6112, 0.7939, 0.9270, 1.0775, 0.9577, 1.0497, 1.0635]  ExtrapMethod=Clip  UseLastTableValue=on  InternalRulePriority=Speed  RndMeth=Simplest
  CMTable : Lookup_n-D  NumberOfTableDimensions=1  BreakpointsForDimension1=[0, 2, 4, 6, 8, 10, 12, 14, 16]  Table=[0.0406, 0.0141, -0.0208, -0.0480, -0.2717, -0.4096, -0.1448, -0.2067, -0.2548]  ExtrapMethod=Clip  UseLastTableValue=on  InternalRulePriority=Speed  RndMeth=Simplest
  ClFunction : Subsystem
  CmFunction : Subsystem
  CnFunction : Subsystem
  Constant : Constant  Value=S
  Constant1 : Constant  Value=S
  Constant3 : Constant  Value=0
  Constant4 : Constant  Value=0
  CyFunction : Subsystem
  Degrees to Radians1 : simulink_extras/Transformations/Degrees to Radians
  Dynamic Pressure : aerolibasang/Dynamic Pressure
  Flat Earth to LLA : aerolibtransform2/Flat Earth to LLA  units=Metric (MKS)  ptype=Earth (WGS84)  F=1/298.257223563  R=6378137  refPosPort=off  LL0=[0 10]  psi=0
  Gain : Gain  Gain=-1
  Gain1 : Gain  Gain=-1
  ISA Atmosphere Model : aerolibatmos2/ISA Atmosphere Model  custom=off  g=9.80665  gamma=1.4  R=287.0531  L=0.0065  h_trop=11000  h_strat=20000  rho0=1.225  P0=101325  T0=288.15  h0=0
  "Incidence, Sideslip, & Airspeed" : aerolibasang/Incidence, Sideslip, & Airspeed
  IsNaN : RelationalOperator  Operator=isNaN  OutDataTypeStr=boolean  RndMeth=Simplest  InputSameDT=off
  Mux : Mux  Inputs=3
  Mux1 : Mux  Inputs=3
  Product : Product  Inputs=3
  Product1 : Product  Inputs=3
  Radians to Degrees : simulink_extras/Transformations/Radians to Degrees
  Radians to Degrees1 : simulink_extras/Transformations/Radians to Degrees
  Scope{1..5} (5 alike) : Scope
  Sum4 : Sum  Inputs=-+|  InputSameDT=on  SaturateOnIntegerOverflow=on  OutDataTypeStr=Inherit: Same as first input
  Switch : Switch  Criteria=u2 ~= 0  SaturateOnIntegerOverflow=off  InputSameDT=off
  Terminator{,1..4} (5 alike) : Terminator
  ForceFuselage : Outport
  MomentFuselage : Outport  Port=2
  Altitude : Outport  Port=3
  AOA : Outport  Port=4
  wires:
  "Incidence, Sideslip, & Airspeed"/1 -> AOA/1, Radians to Degrees/1
  "Incidence, Sideslip, & Airspeed"/2 -> Radians to Degrees1/1
  Radians to Degrees/1 -> [AOA]
  [AOA] -> Scope3/1, CLTable/1, CMTable/1, CDTable/1
  aileron(rad)/1 -> [Ail]
  elevator(rad)/1 -> [ele]
  rudder(rad)/1 -> [rud]
  ISA Atmosphere Model/4 -> Dynamic Pressure/2
  ISA Atmosphere Model/1 -> Terminator/1
  ISA Atmosphere Model/2 -> Terminator1/1
  ISA Atmosphere Model/3 -> Terminator2/1
  CDTable/1 -> [CD]
  Dynamic Pressure/1 -> [DP]
  [DP] -> Product/1
  Constant/1 -> Product/2
  [CD] -> Scope1/1, Product/3
  CLTable/1 -> [CL]
  CMTable/1 -> [CM]
  [CL] -> Scope2/1, Product1/3
  Constant1/1 -> Product1/2
  [DP] -> Product1/1
  Product/1 -> Gain/1
  Mux/1 -> ForceFuselage/1
  Gain/1 -> Mux/1
  Product1/1 -> Gain1/1
  Xe(m)/1 -> Flat Earth to LLA/1
  Flat Earth to LLA/2 -> Altitude/1, ISA Atmosphere Model/1
  Flat Earth to LLA/1 -> Terminator3/1
  Constant3/1 -> Flat Earth to LLA/2
  [CM] -> CmFunction/1(Cm)
  [ele] -> CmFunction/4(Ele)
  Angularate/1 -> [AngularRate]
  [AngularRate] -> ClFunction/1(AngularRate)
  [Ail] -> ClFunction/3(Ail)
  [AOS] -> ClFunction/2(AOS)
  [AngularRate] -> CnFunction/1(AngularRate)
  [AOS] -> CnFunction/2(AOS)
  [rud] -> CnFunction/3(rud)
  [Vb] -> Dynamic Pressure/1
  "Incidence, Sideslip, & Airspeed"/3 -> Terminator4/1
  Radians to Degrees1/1 -> Switch/3, IsNaN/1
  IsNaN/1 -> Switch/2
  Constant4/1 -> Switch/1
  Sum4/1 -> [Vb], "Incidence, Sideslip, & Airspeed"/1
  Wind_V/1 -> Sum4/1
  Gain1/1 -> Mux/3
  Vb(m/s)/1 -> Sum4/2
  Switch/1 -> Degrees to Radians1/1, Scope4/1
  Degrees to Radians1/1 -> [AOS]
  Mux1/1 -> MomentFuselage/1
  [DP] -> ClFunction/5(DP)
  [rud] -> ClFunction/4(Rud)
  [DP] -> CnFunction/5(DP)
  [Ail] -> CnFunction/4(Ail)
  CyFunction/1(y force) -> Mux/2
  [AngularRate] -> CyFunction/1(AngularRate)
  [AOS] -> CyFunction/2(AOS)
  [rud] -> CyFunction/3(Rud)
  [DP] -> CyFunction/4(DP)
  [DP] -> CmFunction/3(DP)
  [Ail] -> CmFunction/2(Ail)
  ClFunction/1(RollMoment) -> Mux1/1
  CmFunction/1(PitchMoment) -> Mux1/2
  CnFunction/1(YawMoment) -> Scope5/1, Mux1/3  "yaw moment"

== system LC62_PIDControl_V6/System Dynamics (LC62-50B)/LC62-50BModel/GravityForce ==
  In1 : Inport
  In2 : Inport  Port=2
  Constant3 : Constant  Value=0
  Flat Earth to LLA : aerolibtransform2/Flat Earth to LLA  units=Metric (MKS)  ptype=Earth (WGS84)  F=1/298.257223563  R=6378137  refPosPort=off  LL0=[0 10]  psi=0
  Gravity in Earth Axes : Gain  Gain=m  SaturateOnIntegerOverflow=on  OutDataTypeStr=Inherit: Same as input  ParamDataTypeStr=Inherit: Same as input
  Inertial to Body : Product  Multiplication=Matrix(*)  InputSameDT=on  SaturateOnIntegerOverflow=on  OutDataTypeStr=Inherit: Same as first input
  Mux : Mux  Inputs=2
  Reshape : Reshape  OutputDimensionality=Column vector (2-D)
  "WGS84 Gravity Model  " : GravityWGS84
  Out1 : Outport
  wires:
  Reshape/1 -> Inertial to Body/2
  In1/1 -> Inertial to Body/1
  Constant3/1 -> Flat Earth to LLA/2
  In2/1 -> Flat Earth to LLA/1
  Flat Earth to LLA/1 -> Mux/1
  Flat Earth to LLA/2 -> Mux/2
  Mux/1 -> "WGS84 Gravity Model  "/1
  "WGS84 Gravity Model  "/1 -> Gravity in Earth Axes/1
  Gravity in Earth Axes/1 -> Reshape/1
  Inertial to Body/1 -> Out1/1

== system LC62_PIDControl_V6/System Dynamics (LC62-50B)/LC62-50BModel/Pusher ==
  PWMInput(1000~2000) : Inport
  Add : Sum
  Add1 : Sum
  Constant : Constant  Value=0
  Constant1 : Constant  Value=0
  Demux : Demux  Outputs=2
  Gain : Gain  Gain=-1
  Mux : Mux  Inputs=3
  Mux1 : Mux  Inputs=3
  Rotor01 : Subsystem
  Rotor02 : Subsystem
  Force : Outport
  Moment : Outport  Port=2
  wires:
  Gain/1 -> Add1/2
  Mux1/1 -> Moment/1
  Add1/1 -> Mux1/1
  Constant1/1 -> Mux1/2, Mux1/3
  [Torque2] -> Gain/1
  [Torque1] -> Add1/1
  [Thrust2] -> Add/2
  Rotor02/2(Torque) -> [Torque2]
  Rotor02/1(Thrust) -> [Thrust2]
  [Thrust1] -> Add/1
  Rotor01/2(Torque) -> [Torque1]
  Rotor01/1(Thrust) -> [Thrust1]
  Constant/1 -> Mux/2, Mux/3
  Mux/1 -> Force/1
  [PWM2] -> Rotor02/1(In1)
  [PWM1] -> Rotor01/1(In1)
  Demux/2 -> [PWM2]
  Demux/1 -> [PWM1]
  PWMInput(1000~2000)/1 -> Demux/1
  Add/1 -> Mux/1

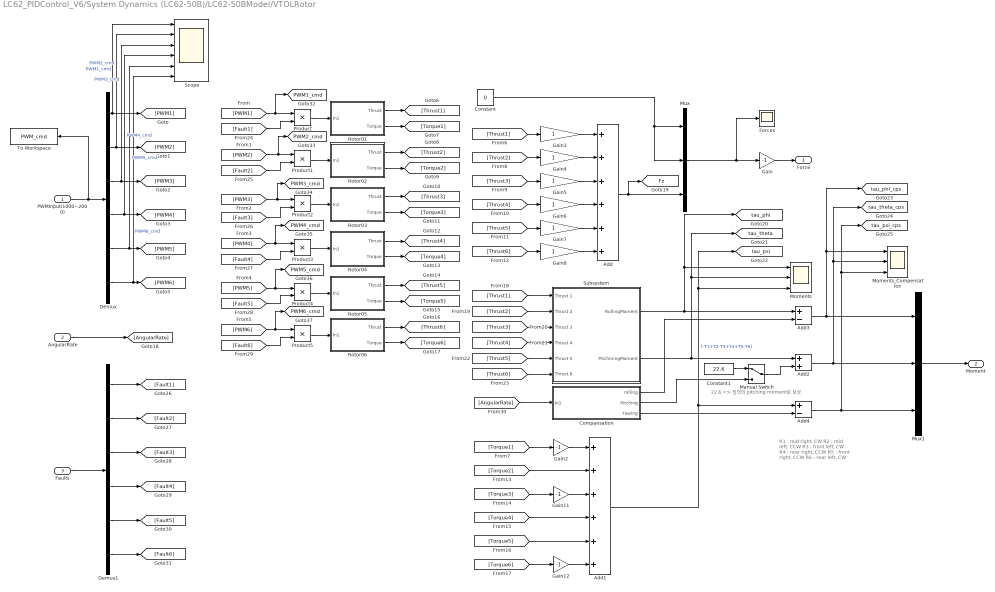
== system LC62_PIDControl_V6/System Dynamics (LC62-50B)/LC62-50BModel/VTOLRotor ==
  note: 22.6 => 임의의 pitching moment로 보상
  note: R1 : mid right, CW
      | R2 : mid left, CCW
      | R3 : front left, CW
      | R4 : rear right, CCW
      | R5 : front right, CCW
      | R6 : rear left, CW
  PWMInput(1000~2000) : Inport
  AngularRate : Inport  Port=2
  Faults : Inport  Port=3
  Add : Sum  Inputs=++++++
  Add1 : Sum  Inputs=++++++
  Add2 : Sum
  Add3 : Sum  Inputs=+-
  Add4 : Sum  Inputs=+-
  Compansation : Subsystem
  Constant : Constant  Value=0
  Constant1 : Constant  Value=22.6
  Demux : Demux  Outputs=6
  Demux1 : Demux  Outputs=6
  Forces : Scope
  Gain{,2,11..12} (4 alike) : Gain  Gain=-1
  Gain{3..8} (6 alike) : Gain
  Manual Switch : ManualSwitch
  Moments : Scope  NumInputPorts=3
  Moments_Compensation : Scope  NumInputPorts=3
  Mux : Mux  Inputs=3
  Mux1 : Mux  Inputs=3
  Product{,1..5} (6 alike) : Product
  Rotor01 : Subsystem
  Rotor02 : Subsystem
  Rotor03 : Subsystem
  Rotor04 : Subsystem
  Rotor05 : Subsystem
  Rotor06 : Subsystem
  Scope : Scope  NumInputPorts=6
  Subsystem : Subsystem
  To Workspace : ToWorkspace  VariableName=PWM_cmd  SaveFormat=Timeseries  SampleTime=-1
  Force : Outport
  Moment : Outport  Port=2
  tag scope: Fz=global, PWM1_cmd=global, PWM2_cmd=global, PWM3_cmd=global, PWM4_cmd=global, PWM5_cmd=global, PWM6_cmd=global, tau_phi=global, tau_phi_cps=global, tau_psi=global, tau_psi_cps=global, tau_theta=global, tau_theta_cps=global
  wires:
  PWMInput(1000~2000)/1 -> To Workspace/1, Demux/1
  Demux/1 -> [PWM1], Scope/1  "PWM1_cmd"
  Demux/2 -> [PWM2], Scope/2  "PWM2_cmd"
  Demux/4 -> [PWM4], Scope/4  "PWM4_cmd"
  Demux/6 -> [PWM6], Scope/6  "PWM6_cmd"
  Constant/1 -> Mux/2, Mux/1
  Add/1 -> Mux/3, [Fz]
  Rotor01/1(Thrust) -> [Thrust1]
  Rotor01/2(Torque) -> [Torque1]
  [Thrust1] -> Gain3/1
  Rotor02/1(Thrust) -> [Thrust2]
  Rotor02/2(Torque) -> [Torque2]
  Rotor03/1(Thrust) -> [Thrust3]
  Rotor03/2(Torque) -> [Torque3]
  Rotor04/1(Thrust) -> [Thrust4]
  Rotor04/2(Torque) -> [Torque4]
  Rotor05/1(Thrust) -> [Thrust5]
  Rotor05/2(Torque) -> [Torque5]
  Rotor06/1(Thrust) -> [Thrust6]
  Rotor06/2(Torque) -> [Torque6]
  [Thrust2] -> Gain4/1
  [Thrust3] -> Gain5/1
  [Thrust4] -> Gain6/1
  [Thrust5] -> Gain7/1
  [Thrust6] -> Gain8/1
  [Thrust1] -> Subsystem/1(Thrust 1)
  [Thrust2] -> Subsystem/2(Thrust 2)
  [Thrust3] -> Subsystem/3(Thrust 3)
  [Thrust4] -> Subsystem/4(Thrust 4)
  [Thrust5] -> Subsystem/5(Thrust 5)
  [Thrust6] -> Subsystem/6(Thrust 6)
  Demux/3 -> [PWM3], Scope/3  "PWM3_cmd"
  Demux/5 -> [PWM5], Scope/5  "PWM5_cmd"
  Subsystem/1(RollingMoment) -> Add3/1, [tau_phi], Moments/1
  AngularRate/1 -> [AngularRate]
  Subsystem/2(PitchmingMoment) -> Add2/1, [tau_theta], Moments/2
  [AngularRate] -> Compansation/1(In1)
  Add3/1 -> [tau_phi_cps], Moments_Compensation/1, Mux1/1
  Add1/1 -> Moments/3, [tau_psi], Add4/1  "(-T1+T2-T3+T4+T5-T6)"
  Compansation/1(rolling) -> Add3/2
  Compansation/3(Yawing) -> Add4/2
  Mux1/1 -> Moment/1
  Add2/1 -> Mux1/2, [tau_theta_cps], Moments_Compensation/2
  Add4/1 -> [tau_psi_cps], Moments_Compensation/3, Mux1/3
  [Torque1] -> Gain2/1
  [Torque3] -> Gain11/1
  [Torque6] -> Gain12/1
  Gain3/1 -> Add/1
  Gain4/1 -> Add/2
  Gain5/1 -> Add/3
  Gain6/1 -> Add/4
  Gain7/1 -> Add/5
  Gain8/1 -> Add/6
  [Torque2] -> Add1/2
  [Torque4] -> Add1/4
  [Torque5] -> Add1/5
  Compansation/2(Pitching) -> Manual Switch/2
  Mux/1 -> Forces/1, Gain/1
  Gain/1 -> Force/1
  Gain2/1 -> Add1/1
  Gain11/1 -> Add1/3
  Gain12/1 -> Add1/6
  Manual Switch/1 -> Add2/2
  Constant1/1 -> Manual Switch/1
  [PWM1] -> [PWM1_cmd], Product/1
  Product/1 -> Rotor01/1(In1)
  Product1/1 -> Rotor02/1(In1)
  [PWM2] -> [PWM2_cmd], Product1/1
  Product2/1 -> Rotor03/1(In1)
  [PWM3] -> [PWM3_cmd], Product2/1
  Product3/1 -> Rotor04/1(In1)
  [PWM4] -> [PWM4_cmd], Product3/1
  [PWM5] -> [PWM5_cmd], Product4/1
  Product4/1 -> Rotor05/1(In1)
  Product5/1 -> Rotor06/1(In1)
  [PWM6] -> [PWM6_cmd], Product5/1
  Demux1/5 -> [Fault5]
  Demux1/3 -> [Fault3]
  Demux1/6 -> [Fault6]
  Demux1/4 -> [Fault4]
  Demux1/2 -> [Fault2]
  Demux1/1 -> [Fault1]
  Faults/1 -> Demux1/1
  [Fault1] -> Product/2
  [Fault2] -> Product1/2
  [Fault3] -> Product2/2
  [Fault4] -> Product3/2
  [Fault5] -> Product4/2
  [Fault6] -> Product5/2

== system LC62_PIDControl_V6/System Dynamics (LC62-50B)/LC62-50BModel/WindModel ==
  Ve : Inport  Unit=m/s
  Altitude : Inport  Port=2  Unit=meter
  DCM : Inport  Port=3
  Discrete Wind Gust Model1 : aerolibwind2/Discrete Wind Gust Model  units=Metric (MKS)  Gx=off  Gy=off  Gz=off  t_0=20  d_m=[120 120 80]  v_m=[5, 5, 5]
  Dot Product : DotProduct  OutDataTypeStr=Inherit: Inherit via internal rule
  Dryden Wind Turbulence Model (Discrete (+q -r)) : aerolibwind2/Dryden Wind Turbulence Model  (Continuous (+q -r))  units=Metric (MKS)  spec=MIL-F-8785C  model=Discrete Dryden (+q -r)  W20=5  Wdeg=0  TurbProb=10^-2 - Light  L_high=533.4  Wingspan=4  ts=0.1  Seed=[23341 23342 23343 23344]  T_on=on
  Mux : Mux  Inputs=2
  Sqrt : Sqrt
  Sum : Sum  Inputs=+++  InputSameDT=on  SaturateOnIntegerOverflow=on  OutDataTypeStr=Inherit: Same as first input
  Wind Shear Model1 : aerolibwind2/Wind Shear Model  units=Metric (MKS)  phase=Category C - Terminal Flight Phase  W_20=5  Wdeg=0
  ug,vg,wg,pg,qg,wg : Outport  Unit=m/s  VectorParamsAs1DForOutWhenUnconnected=off
  wires:
  Altitude/1 -> Dryden Wind Turbulence Model (Discrete (+q -r))/1, Wind Shear Model1/1
  DCM/1 -> Dryden Wind Turbulence Model (Discrete (+q -r))/3, Wind Shear Model1/2
  Discrete Wind Gust Model1/1 -> Sum/3
  Wind Shear Model1/1 -> Sum/1
  Dryden Wind Turbulence Model (Discrete (+q -r))/1 -> Sum/2
  Dot Product/1 -> Sqrt/1
  Ve/1 -> Dot Product/1, Dot Product/2
  Sqrt/1 -> Discrete Wind Gust Model1/1, Dryden Wind Turbulence Model (Discrete (+q -r))/2
  Mux/1 -> ug,vg,wg,pg,qg,wg/1
  Sum/1 -> Mux/1
  Dryden Wind Turbulence Model (Discrete (+q -r))/2 -> Mux/2

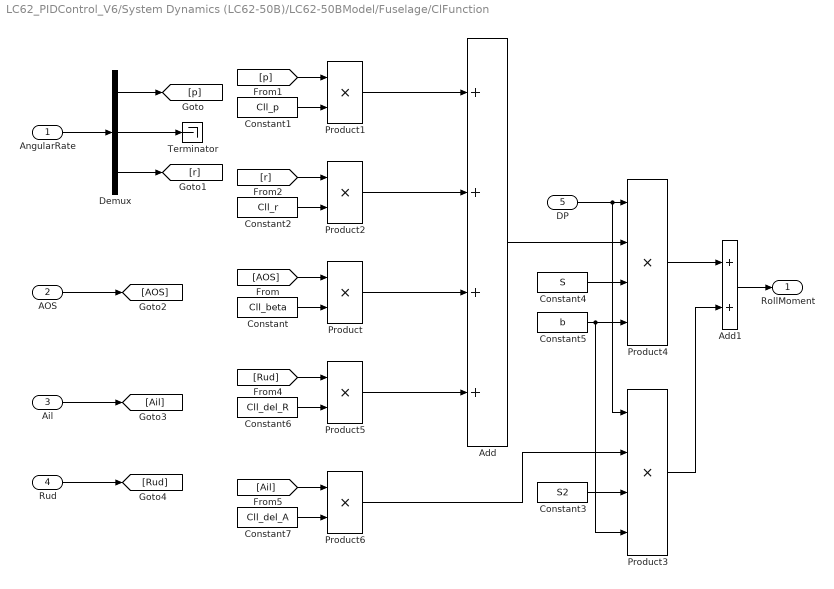
== system LC62_PIDControl_V6/System Dynamics (LC62-50B)/LC62-50BModel/Fuselage/ClFunction ==
  AngularRate : Inport
  AOS : Inport  Port=2
  Ail : Inport  Port=3
  Rud : Inport  Port=4
  DP : Inport  Port=5
  Add : Sum  Inputs=++++
  Add1 : Sum
  Constant : Constant  Value=Cll_beta
  Constant1 : Constant  Value=Cll_p
  Constant2 : Constant  Value=Cll_r
  Constant3 : Constant  Value=S2
  Constant4 : Constant  Value=S
  Constant5 : Constant  Value=b
  Constant6 : Constant  Value=Cll_del_R
  Constant7 : Constant  Value=Cll_del_A
  Demux : Demux  Outputs=3
  Product{,1..2,5..6} (5 alike) : Product
  Product3 : Product  Inputs=4
  Product4 : Product  Inputs=4
  Terminator : Terminator
  RollMoment : Outport
  wires:
  AngularRate/1 -> Demux/1
  Demux/1 -> [p]
  Demux/3 -> [r]
  Demux/2 -> Terminator/1
  AOS/1 -> [AOS]
  Ail/1 -> [Ail]
  [AOS] -> Product/1
  Constant/1 -> Product/2
  Constant1/1 -> Product1/2
  [p] -> Product1/1
  [r] -> Product2/1
  Constant2/1 -> Product2/2
  Product/1 -> Add/3
  Product2/1 -> Add/2
  Product1/1 -> Add/1
  Add/1 -> Product4/2
  Constant4/1 -> Product4/3
  Constant5/1 -> Product3/4, Product4/4
  Product5/1 -> Add/4
  Constant6/1 -> Product5/2
  [Rud] -> Product5/1
  Rud/1 -> [Rud]
  DP/1 -> Product3/1, Product4/1
  Constant7/1 -> Product6/2
  [Ail] -> Product6/1
  Product4/1 -> Add1/1
  Add1/1 -> RollMoment/1
  Product6/1 -> Product3/2
  Constant3/1 -> Product3/3
  Product3/1 -> Add1/2

== system LC62_PIDControl_V6/System Dynamics (LC62-50B)/LC62-50BModel/Fuselage/CmFunction ==
  Cm : Inport
  Ail : Inport  Port=2
  DP : Inport  Port=3
  Ele : Inport  Port=4
  Add : Sum  Inputs=+++
  Cm_del_A : Constant  Value=Cm_del_A
  Cm_del_E : Constant  Value=Cm_del_E
  Constant4 : Constant  Value=S
  Constant5 : Constant  Value=c
  Product1 : Product
  Product3 : Product  Inputs=4
  Product4 : Product
  PitchMoment : Outport
  wires:
  Product3/1 -> PitchMoment/1
  Cm/1 -> Add/1
  Constant5/1 -> Product3/2
  Constant4/1 -> Product3/1
  Add/1 -> Product3/3
  Cm_del_A/1 -> Product1/2
  Ail/1 -> Product1/1
  DP/1 -> Product3/4
  Product1/1 -> Add/3
  Ele/1 -> Product4/1
  Product4/1 -> Add/2
  Cm_del_E/1 -> Product4/2
